simulink model "zbiornik_sys"  (R2024b)
settings: Solver=VariableStepAuto  StartTime=0.0  StopTime=10.0  RelTol=1e-3
settings Model: Creator=student  LastModifiedBy=adasf

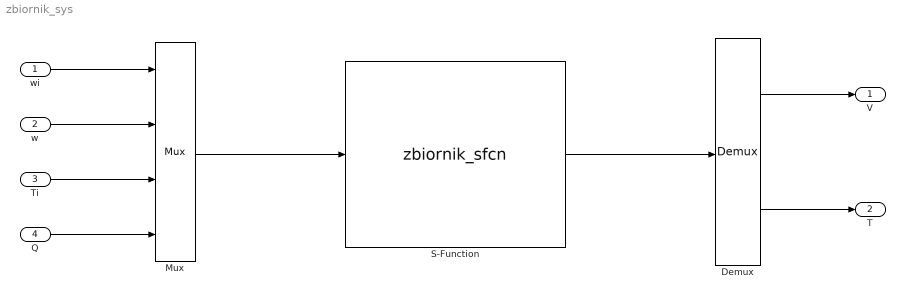
== system zbiornik_sys ==
  wi : Inport
  w : Inport  Port=2
  Ti : Inport  Port=3
  Q : Inport  Port=4
  Demux : Demux  Outputs=2
  Mux : Mux
  S-Function : S-Function  FunctionName=zbiornik_sfcn  Parameters=V0 T0  SFunctionDeploymentMode=off  EnableBusSupport=off
  V : Outport
  T : Outport  Port=2
  wires:
  wi/1 -> Mux/1
  w/1 -> Mux/2
  Ti/1 -> Mux/3
  Q/1 -> Mux/4
  Mux/1 -> S-Function/1
  S-Function/1 -> Demux/1
  Demux/2 -> T/1
  Demux/1 -> V/1
